simulink model "VInoLineal"  (R2021a)
settings: Solver=FixedStepAuto  StartTime=0.0  StopTime=10.0  FixedStep=T  RelTol=1e-3
values from neighbouring files (symbols this model uses):
  T = 0.05    [CompensatorDesignToolbox.m]
libraries: cstblocks x3, simulink x2
settings Model: Creator=MarcosRPesanteColón  LastModifiedBy=MarcosRPesanteColón

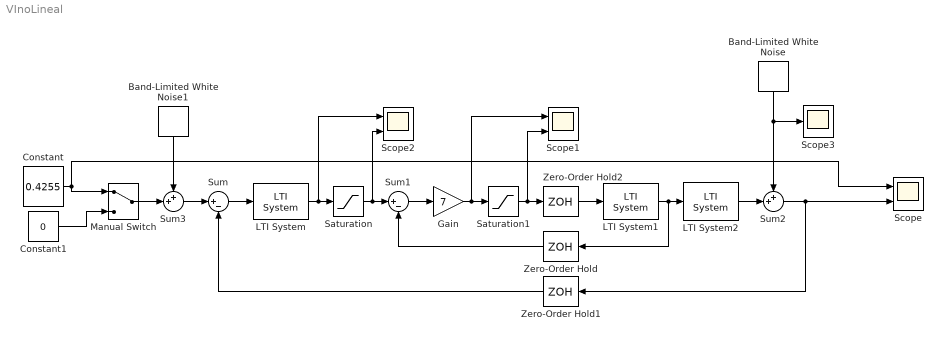
== system VInoLineal ==
  Band-Limited White Noise : simulink/Sources/Band-Limited White Noise  Cov=1E-6  Ts=T  seed=[23341]
  Band-Limited White Noise1 : simulink/Sources/Band-Limited White Noise  Cov=1E-6  Ts=T  seed=[23341]
  Constant : Constant  Value=0.4255
  Constant1 : Constant  Value=0
  Gain : Gain  Gain=7
  LTI System : cstblocks/LTI System  sys=tmp  IC=[]
  LTI System1 : cstblocks/LTI System  sys=G_m  IC=[]
  LTI System2 : cstblocks/LTI System  sys=G_bb  IC=[]
  Manual Switch : ManualSwitch
  Saturation : Saturate  UpperLimit=pi/2  LowerLimit=-pi/2
  Saturation1 : Saturate  UpperLimit=5  LowerLimit=-5
  Scope : Scope  NumInputPorts=2
  Scope1 : Scope  NumInputPorts=2
  Scope2 : Scope  NumInputPorts=2
  Scope3 : Scope
  Sum : Sum  Inputs=|+-
  Sum1 : Sum  Inputs=|+-
  Sum2 : Sum  Inputs=++|
  Sum3 : Sum  Inputs=++|
  Zero-Order Hold : ZeroOrderHold  SampleTime=-1
  Zero-Order Hold1 : ZeroOrderHold  SampleTime=-1
  Zero-Order Hold2 : ZeroOrderHold  SampleTime=-1
  wires:
  Constant1/1 -> Manual Switch/2
  Constant/1 -> Scope/1, Manual Switch/1
  Sum/1 -> LTI System/1
  LTI System/1 -> Scope2/1, Saturation/1
  Saturation/1 -> Scope2/2, Sum1/1
  Sum1/1 -> Gain/1
  Gain/1 -> Scope1/1, Saturation1/1
  Saturation1/1 -> Scope1/2, Zero-Order Hold2/1
  LTI System1/1 -> Zero-Order Hold/1, LTI System2/1
  Zero-Order Hold/1 -> Sum1/2
  Zero-Order Hold1/1 -> Sum/2
  Zero-Order Hold2/1 -> LTI System1/1
  LTI System2/1 -> Sum2/2
  Sum2/1 -> Zero-Order Hold1/1, Scope/2
  Band-Limited White Noise/1 -> Sum2/1, Scope3/1
  Sum3/1 -> Sum/1
  Manual Switch/1 -> Sum3/2
  Band-Limited White Noise1/1 -> Sum3/1
